simulink model "Model_TranslationEngine64"  (R2022b)
settings: Solver=FixedStepDiscrete  StartTime=0.0  StopTime=5  RelTol=1e-3  EnableMultiTasking=on
InitFcn:
  | % Initialize model
  | ModelSettings=BTConfig.GetModelSettings();
  | 
  | ModelSettings.Validate();
  | 
  | ModelInit;
  | 
  | 
  | % load library data
  | GainLibrary_data;
  | % Load saved values from partition process
  | CapturedConstMask.LoadMapFromFile(bdroot)
StartFcn:
  | % make sure all the simulated RTC requests are found
  | %RTC_SIM_OBJ.ValidateREQs();
undefined symbols (not defined in the file or in its folder): AA, BPLP, Column, NumHFRefBPF, NumHFRefLPF, NumMusicChannels, Row, VolumeMuteConfig
libraries: TuneVar x925, TOP x490, FeaturePath x111, CapturedConstLib x52
(part 14 of 34)

== system Model_TranslationEngine64/ModelPreAmp/DecRate/Medusa5H1/SleepingBeauty/SleepingBeauty/Enabled ==
  FadeControl : Subsystem  mask(Bose FadeControl){MaskIndexOffset=128, MaskBoostDisable=off, MaskSilentExtreme=on, BankNumber=0}
      mask prompts: MaskIndexOffset "Index Offset"; MaskBoostDisable "Disable Boost"; MaskSilentExtreme "Enable Silent Extreme"; BankNumber "Target Memory Bank Number"
      mask help: This component is to be used in conjunction with 1 or more instances of the FadeRamper block. It provides the control layer for Fade processing via an RTC and tune variables.
      mask init:
      | blkh = gcbh;
      | % Copy discrete mask parameters into a classdef object
      | InnerLinkConfig = FadeControlConfig;
      | InnerLinkConfig.DefaultIndexOffset = MaskIndexOffset;
      | InnerLinkConfig.DefaultBoostDisable = MaskBoostDisable;
      | InnerLinkConfig.DefaultSilentExtreme = MaskSilentExtreme;
      | InnerLinkConfig.BankNumber = BankNumber;
      mask Help: If this control block is being used in a "multi-instance" manner, i.e. it is contorlling two or more FadeRamper blocks, there is an additional step that must be done. The developer must add a function-triggered subsytem containing an AND logic gate, which will combine the notification completion signals of the multiple ramper instances. The output of this subsytem must then feed the NTF_done input of the FadeControl block.
  FadeRamperDR : Subsystem  mask(Bose FadeRamper){MaskFeatureName=FadeRamperDR, MaskChanRampMap=ones(1,30), MaskEnableGainPort=on}
      mask prompts: MaskFeatureName "Instance Name"; MaskChanRampMap "Channel to Ramper Map"; MaskEnableGainPort "Enable Output Gain Port"
      mask help:
      | This component is to be used in conjunction with the FadeControl block, which provides runtime control and tuning capabilities. Multiple instances of this block may be placed within an audio application, and a single FadeControl block has the ability to control all of these rampers simultaneously.
      |
      | For "Instance Name", please enter a name for the block. For example, if this is one of multiple instances of FadeRamper, then name each block accordingly so that the subsequent tune variables will route correctly.
      |
      | i.e. FadeRamper1, FadeRamper2, FadeRamperFullRate, etc.
      mask init:
      | blkh = gcbh;
      | % Copy discrete mask parameters into a classdef object
      | InnerLinkConfig = FadeRamperConfig;
      | InnerLinkConfig.DefaultChanRampMap = MaskChanRampMap;
      | 
      | % handle configurable output
      | EnableBlockPort(blkh,'fadeGains',MaskEnableGainPort,'2');
      mask TypeOptions MaskFeatureName: InnerLink/FeatureName
  FadeRamperFR : Subsystem  mask(Bose FadeRamper){MaskFeatureName=FadeRamperFR, MaskChanRampMap=ones(1,22), MaskEnableGainPort=on}
      mask prompts: MaskFeatureName "Instance Name"; MaskChanRampMap "Channel to Ramper Map"; MaskEnableGainPort "Enable Output Gain Port"
      mask help:
      | This component is to be used in conjunction with the FadeControl block, which provides runtime control and tuning capabilities. Multiple instances of this block may be placed within an audio application, and a single FadeControl block has the ability to control all of these rampers simultaneously.
      |
      | For "Instance Name", please enter a name for the block. For example, if this is one of multiple instances of FadeRamper, then name each block accordingly so that the subsequent tune variables will route correctly.
      |
      | i.e. FadeRamper1, FadeRamper2, FadeRamperFullRate, etc.
      mask init: same as Model_TranslationEngine64/ModelPreAmp/DecRate/Medusa5H1/SleepingBeauty/SleepingBeauty/Enabled/FadeRamperDR
      mask TypeOptions MaskFeatureName: InnerLink/FeatureName
  MuteControl : Subsystem  mask(Bose MuteControl){}
      mask help: This component is to be used in conjunction with 1 or more instances of the MuteRamper block. There is no mask for this component. It provides the control layer for Mute processing via an RTC and tune variable, muteControlRampTime.
      mask init:
      | InnerLinkConfig = MuteControlConfig;
      mask Help: If this control block is being used in a "multi-instance" manner, i.e. it is contorlling two or more MuteRamper blocks, there is an additional step that must be done. The developer must add a function-triggered subsytem containing an AND logic gate, which will combine the notification completion signals of the multiple ramper instances. The output of this subsytem must then feed the NTF_done input of the MuteControl block.
  SleepingBeautyDR : Subsystem  mask(Bose SleepingBeauty){MaskFeatureName=SleepingBeautyDR, MaskChanRampMap=ones(1,30), MaskOffset=128, MaskSilentExtremeMutesBass=off}
      mask prompts: MaskFeatureName "Instance Name"; MaskChanRampMap "Channel to Ramper Map"; MaskOffset "Control Index Offset"; MaskSilentExtremeMutesBass "Silent Extreme Mutes Bass"
      mask help:
      | This block is to be used in conjunction with the Balance block.
      |
      | For the Channel to Ramper Map, enter any of the following values:
      | 1 - left channel
      | 2 - right channel
      | 3 - center channel
      | 4 - mono channel
      | -1 - unused channel (will esentially be muted)
      | (For headrest speakers, choose a seat-centric ramper, i.e. Left Seat Left Ear and Left Seat Right Ear would both be considered "Left content", receiving a 1).
      |
      | Silent Extreme Mutes Bass: Check this box if the intention is for mono channels to be muted upon Silent Extreme
      |
      | If this block is being used in a multi-instance application, be sure to give independent names in each instance's mask.
      mask init:
      | blkh = gcbh;
      | % Copy discrete mask parameters into a classdef object
      | InnerLinkConfig = SleepingBeautyConfig;
      | InnerLinkConfig.ChanToRampMap = MaskChanRampMap;
      | InnerLinkConfig.DefaultOffset = MaskOffset;
      | InnerLinkConfig.DefaultSilentExtremeMutesBass = MaskSilentExtremeMutesBass;
      mask TypeOptions MaskFeatureName: InnerLink/FeatureName
  SleepingBeautyFR : Subsystem  mask(Bose SleepingBeauty){MaskFeatureName=SleepingBeautyFR, MaskChanRampMap=ones(1,22), MaskOffset=128, MaskSilentExtremeMutesBass=off}
      mask prompts: MaskFeatureName "Instance Name"; MaskChanRampMap "Channel to Ramper Map"; MaskOffset "Control Index Offset"; MaskSilentExtremeMutesBass "Silent Extreme Mutes Bass"
      mask help:
      | This block is to be used in conjunction with the Balance block.
      |
      | For the Channel to Ramper Map, enter any of the following values:
      | 1 - left channel
      | 2 - right channel
      | 3 - center channel
      | 4 - mono channel
      | -1 - unused channel (will esentially be muted)
      | (For headrest speakers, choose a seat-centric ramper, i.e. Left Seat Left Ear and Left Seat Right Ear would both be considered "Left content", receiving a 1).
      |
      | Silent Extreme Mutes Bass: Check this box if the intention is for mono channels to be muted upon Silent Extreme
      |
      | If this block is being used in a multi-instance application, be sure to give independent names in each instance's mask.
      mask init: same as Model_TranslationEngine64/ModelPreAmp/DecRate/Medusa5H1/SleepingBeauty/SleepingBeauty/Enabled/SleepingBeautyDR
      mask TypeOptions MaskFeatureName: InnerLink/FeatureName

== system Model_TranslationEngine64/ModelPreAmp/DecRate/Medusa5H1/VLS/Crosstalk Cancellation/Pooliir with Non-Trivial Translations ==
  InnerLink : Subsystem  mask(Bose Pool IIR Tunable){FeatureName=IIR, Config=InnerLinkConfig}
      mask prompts: FeatureName "Filter name/purpose"; Config "PoolIirTunableConfig"
      mask help:
      | Pool IIR Tunable is a configurable multi-channel IIR filter that supports one or more channels. This block offers flexibility of tuning the number of stages and coefficients. Different filter coefficients and number of stages (biquads) can be used for each channel filter. The Pool IIR Tunable block supports different implementations, which could be configured at build-time:
      |
      | (i)   Generic: IIR filter code not optimized for any processor
      | (ii)  SharcCore: IIR filters executing on core (uses pooliir.asm CRL)
      | (iii) SharcGulAccel: IIR filters executing on IIR hardware accelerator, offloading MIPS usage from core
      | (iv) SharcGxpAccel: IIR filters take advantage of additional accelerators available on GXP processor
      | (v)  Hexagon: TBD
      |
      | NOTE: When using Pool IIR for Sharc-plus based processors, the codeWorkMemory buffer and input buffer should always be mapped to L1 memory to optimize MIPS utilization and avoid audio artifacts.
      |
      | For more information, please see 'Help'.
      mask init:
      | blkh=gcbh;
      | Config=BTConfig.Assert(blkh,Config);
      | 
      | Config.Validate();
      | Config.DoMaskInit(blkh);
      mask Help:
      | <b>Input signals: </b>
      | AudioIn: input channels [frame size x number of channels]
      | 
      | <b>Output signals: </b>
      | AudioOut: output channels [frame size x number of channels]
      | 
      | <b>Mask parameters: </b>
      | PoolIirTunableConfig
      | Filter name/purpose
      mask TypeOptions FeatureName: PoolIirTunableWithReset/FeatureName
      mask Display: DrawPoolIirIcon;

== system Model_TranslationEngine64/ModelPreAmp/DecRate/Medusa5H1/VLS/Crosstalk Cancellation/TuneTOP ==
  TOP : TOP/TOP  TriggerInit=[440 20 585 80]  TopName=Delay  DataTypeOut=int32  BankNumber=BankNumber  PreOverlay=PreOverlay  PostOverlay=PostOverlay  Role=Automatic
      settings: SourceProductName=Bose Talaria
  TrivialTranslation : TuneVar/TrivialTranslation  TriggerInit=[300 28 350 72]
      settings: SourceProductName=Bose Talaria
  Tune Variable : TuneVar/TuneVar  TuneName=Delay  SpecifyMaxSize=off  VariableDim=1 (Row)  MaxSize=[1 1]  TunabilityNumber=1  MinValue=MinValue  MaxValue=MaxValue  TriggerInit=[20 25 190 75]  MaskValue=MaskValue
      settings: SourceProductName=Bose Talaria
  wires:
  Tune Variable/1 -> TrivialTranslation/1  "Delay"
  TrivialTranslation/1 -> TOP/1

== system Model_TranslationEngine64/ModelPreAmp/PreAmpPart1/NEARPreAmp/FixedAttenuator/Attenuation /Function-Call Subsystem ==
  In1 : Inport
  function : TriggerPort  TriggerType=function-call  VariantControl=Variant
  MATLAB Function : MATLAB Function  TreatAsAtomicUnit=on
  Out1 : Outport
  wires:
  MATLAB Function/1(lingain) -> Out1/1
  In1/1 -> MATLAB Function/1(dbgain)

== system Model_TranslationEngine64/ModelPreAmp/PreAmpPart1/NEARPreAmp/Monoizer/Monoizer/MonoizerStereo ==
  MonoizerCalc : Subsystem

== system Model_TranslationEngine64/ModelPreAmp/PreAmpPart1/NEARPreAmp/Monoizer/Monoizer/MonoizerSurround ==

== system Model_TranslationEngine64/NEAR/Near1p1/DrProc/FsEQDr/Pooliir/PoolIirTunableWithReset ==
  CapturedTuneConst : CapturedConstLib/CapturedConst  TriggerInit=[-600 302 -500 338]  Role=Automatic
      settings: SourceProductName=Bose Talaria
  FeaturePath : FeaturePath/FeaturePath  FeatureName=Pooliir  IsGroup=off  GroupNumber=-1  IsModule=off  TriggerInit=[-750 -81 -635 26]
      settings: SourceProductName=Bose Talaria
  TOP : TOP/TOP  TriggerInit=[-145 187 5 243]  TopName=PooliirNumStages  DataTypeOut=uint32  BankNumber=0  PreOverlay=false  PostOverlay=Config.VariantObj.PostOverlayRequired  Role=Automatic
      settings: SourceProductName=Bose Talaria
  TOP1 : TOP/TOP  TriggerInit=[-140 277 10 333]  TopName=pooliirCoeffs  DataTypeOut=single  BankNumber=0  PreOverlay=false  PostOverlay=Config.VariantObj.PostOverlayRequired  Role=Automatic
      settings: SourceProductName=Bose Talaria
  TranslateTrigger : TuneVar/TranslateTrigger  TriggerInit=[-339 35 -301 90]
      settings: SourceProductName=Bose Talaria
  Translation : MATLAB Function  TreatAsAtomicUnit=on  mask{MaxNumStages=Config.MaxNumStages, VariantUint8=Config.Variant.Uint8Str}
      mask prompts: VariantUint8 "Variant"
  Tune Variable1 : TuneVar/TuneVar  TuneName=numStages  SpecifyMaxSize=off  VariableDim=1 (Row)  MaxSize=[1 1]  TunabilityNumber=1  MinValue=[]  MaxValue=[]  TriggerInit=[-750 235 -580 285]  MaskValue=Config.TuneDefaults.NumStages
      settings: SourceProductName=Bose Talaria
  Tune Variable2 : TuneVar/TuneVar  TuneName=sosCoefficients  SpecifyMaxSize=on  VariableDim=1 (Row)  MaxSize=[Config.MaxNumStages 6]  TunabilityNumber=1  MinValue=[]  MaxValue=[]  TriggerInit=[-750 175 -580 225]  MaskValue=Config.TuneDefaults.SosCoefficients
      settings: SourceProductName=Bose Talaria
  wires:
  TranslateTrigger/1 -> Translation/Trigger
  Tune Variable2/1 -> Translation/1(RawSOS)  "sosCoefficients"
  Translation/2(PoolCoeffs) -> TOP1/1
  Translation/1(PoolNumStages) -> TOP/1
  Tune Variable1/1 -> Translation/2(NumStages)  "numStages"
  CapturedTuneConst/1 -> Translation/3(NumChannels)

== system Model_TranslationEngine64/NEAR/Near1p1/DrProc/FsEQDr/Subsystem1/Subsystem ==
  Tune Variable : TuneVar/TuneVar  TuneName=f1_del  SpecifyMaxSize=off  VariableDim=1 (Row)  MaxSize=[1 1]  TunabilityNumber=1  MinValue=[]  MaxValue=[]  TriggerInit=[20 20 190 70]  MaskValue=Config.f1_del
      settings: SourceProductName=Bose Talaria
  Tune Variable1 : TuneVar/TuneVar  TuneName=f2_del  SpecifyMaxSize=off  VariableDim=1 (Row)  MaxSize=[1 1]  TunabilityNumber=1  MinValue=[]  MaxValue=[]  TriggerInit=[20 155 190 205]  MaskValue=Config.f2_del
      settings: SourceProductName=Bose Talaria
  Tune Variable2 : TuneVar/TuneVar  TuneName=f3_del  SpecifyMaxSize=off  VariableDim=1 (Row)  MaxSize=[1 1]  TunabilityNumber=1  MinValue=[]  MaxValue=[]  TriggerInit=[20 290 190 340]  MaskValue=Config.f3_del
      settings: SourceProductName=Bose Talaria
  Tune Variable3 : TuneVar/TuneVar  TuneName=f4_del  SpecifyMaxSize=off  VariableDim=1 (Row)  MaxSize=[1 1]  TunabilityNumber=1  MinValue=[]  MaxValue=[]  TriggerInit=[20 425 190 475]  MaskValue=Config.f4_del
      settings: SourceProductName=Bose Talaria
  Tune Variable4 : TuneVar/TuneVar  TuneName=f5_del  SpecifyMaxSize=off  VariableDim=1 (Row)  MaxSize=[1 1]  TunabilityNumber=1  MinValue=[]  MaxValue=[]  TriggerInit=[20 560 190 610]  MaskValue=Config.f5_del
      settings: SourceProductName=Bose Talaria
  Tune Variable5 : TuneVar/TuneVar  TuneName=f6_del  SpecifyMaxSize=off  VariableDim=1 (Row)  MaxSize=[1 1]  TunabilityNumber=1  MinValue=[]  MaxValue=[]  TriggerInit=[20 695 190 745]  MaskValue=Config.f6_del
      settings: SourceProductName=Bose Talaria
  Tune Variable7 : TuneVar/TuneVar  TuneName=f7_del  SpecifyMaxSize=off  VariableDim=1 (Row)  MaxSize=[1 1]  TunabilityNumber=1  MinValue=[]  MaxValue=[]  TriggerInit=[20 825 190 875]  MaskValue=Config.f7_del
      settings: SourceProductName=Bose Talaria
  f1 : Outport
  f2 : Outport  Port=2
  f3 : Outport  Port=3
  f4 : Outport  Port=4
  f5 : Outport  Port=5
  f6 : Outport  Port=6
  f7 : Outport  Port=7
  wires:
  Tune Variable5/1 -> f6/1  "f6_del"
  Tune Variable2/1 -> f3/1  "f3_del"
  Tune Variable7/1 -> f7/1  "f7_del"
  Tune Variable/1 -> f1/1  "f1_del"
  Tune Variable1/1 -> f2/1  "f2_del"
  Tune Variable3/1 -> f4/1  "f4_del"
  Tune Variable4/1 -> f5/1  "f5_del"

== system Model_TranslationEngine64/NEAR/Near1p1/DrProc/HrEQDr/PoolIirTunable/PoolIirTunableWithReset ==
  CapturedTuneConst : CapturedConstLib/CapturedConst  TriggerInit=[-600 302 -500 338]  Role=Automatic
      settings: SourceProductName=Bose Talaria
  FeaturePath : FeaturePath/FeaturePath  FeatureName=PoolIirTunable  IsGroup=off  GroupNumber=-1  IsModule=off  TriggerInit=[-750 -81 -635 26]
      settings: SourceProductName=Bose Talaria
  TOP : TOP/TOP  TriggerInit=[-145 187 5 243]  TopName=PooliirNumStages  DataTypeOut=uint32  BankNumber=0  PreOverlay=false  PostOverlay=Config.VariantObj.PostOverlayRequired  Role=Automatic
      settings: SourceProductName=Bose Talaria
  TOP1 : TOP/TOP  TriggerInit=[-140 277 10 333]  TopName=pooliirCoeffs  DataTypeOut=single  BankNumber=0  PreOverlay=false  PostOverlay=Config.VariantObj.PostOverlayRequired  Role=Automatic
      settings: SourceProductName=Bose Talaria
  TranslateTrigger : TuneVar/TranslateTrigger  TriggerInit=[-339 35 -301 90]
      settings: SourceProductName=Bose Talaria
  Translation : MATLAB Function  TreatAsAtomicUnit=on  mask{MaxNumStages=Config.MaxNumStages, VariantUint8=Config.Variant.Uint8Str}
      mask prompts: VariantUint8 "Variant"
  Tune Variable1 : TuneVar/TuneVar  TuneName=numStages  SpecifyMaxSize=off  VariableDim=1 (Row)  MaxSize=[1 1]  TunabilityNumber=1  MinValue=[]  MaxValue=[]  TriggerInit=[-750 235 -580 285]  MaskValue=Config.TuneDefaults.NumStages
      settings: SourceProductName=Bose Talaria
  Tune Variable2 : TuneVar/TuneVar  TuneName=sosCoefficients  SpecifyMaxSize=on  VariableDim=1 (Row)  MaxSize=[Config.MaxNumStages 6]  TunabilityNumber=1  MinValue=[]  MaxValue=[]  TriggerInit=[-750 175 -580 225]  MaskValue=Config.TuneDefaults.SosCoefficients
      settings: SourceProductName=Bose Talaria
  wires:
  TranslateTrigger/1 -> Translation/Trigger
  Tune Variable2/1 -> Translation/1(RawSOS)  "sosCoefficients"
  Translation/2(PoolCoeffs) -> TOP1/1
  Translation/1(PoolNumStages) -> TOP/1
  Tune Variable1/1 -> Translation/2(NumStages)  "numStages"
  CapturedTuneConst/1 -> Translation/3(NumChannels)

== system Model_TranslationEngine64/NEAR/Near1p1/DrProc/HrEQDr/Subsystem2/Subsystem ==
  Tune Variable1 : TuneVar/TuneVar  TuneName=driver_src1  SpecifyMaxSize=off  VariableDim=1 (Row)  MaxSize=[1 1]  TunabilityNumber=1  MinValue=[]  MaxValue=[]  TriggerInit=[35 385 205 435]  MaskValue=Config.driver_src1
      settings: SourceProductName=Bose Talaria
  Tune Variable2 : TuneVar/TuneVar  TuneName=driver_src2  SpecifyMaxSize=off  VariableDim=1 (Row)  MaxSize=[1 1]  TunabilityNumber=1  MinValue=[]  MaxValue=[]  TriggerInit=[35 515 205 565]  MaskValue=Config.driver_src2
      settings: SourceProductName=Bose Talaria
  Tune Variable3 : TuneVar/TuneVar  TuneName=driver_src3  SpecifyMaxSize=off  VariableDim=1 (Row)  MaxSize=[1 1]  TunabilityNumber=1  MinValue=[]  MaxValue=[]  TriggerInit=[35 620 205 670]  MaskValue=Config.driver_src3
      settings: SourceProductName=Bose Talaria
  Tune Variable4 : TuneVar/TuneVar  TuneName=driver_src4  SpecifyMaxSize=off  VariableDim=1 (Row)  MaxSize=[1 1]  TunabilityNumber=1  MinValue=[]  MaxValue=[]  TriggerInit=[35 750 205 800]  MaskValue=Config.driver_src4
      settings: SourceProductName=Bose Talaria
  Tune Variable5 : TuneVar/TuneVar  TuneName=passenger_src1  SpecifyMaxSize=off  VariableDim=1 (Row)  MaxSize=[1 1]  TunabilityNumber=1  MinValue=[]  MaxValue=[]  TriggerInit=[35 880 205 930]  MaskValue=Config.passenger_src1
      settings: SourceProductName=Bose Talaria
  Tune Variable6 : TuneVar/TuneVar  TuneName=passenger_src3  SpecifyMaxSize=off  VariableDim=1 (Row)  MaxSize=[1 1]  TunabilityNumber=1  MinValue=[]  MaxValue=[]  TriggerInit=[35 1140 205 1190]  MaskValue=Config.passenger_src3
      settings: SourceProductName=Bose Talaria
  Tune Variable7 : TuneVar/TuneVar  TuneName=passenger_src2  SpecifyMaxSize=off  VariableDim=1 (Row)  MaxSize=[1 1]  TunabilityNumber=1  MinValue=[]  MaxValue=[]  TriggerInit=[35 1010 205 1060]  MaskValue=Config.passenger_src2
      settings: SourceProductName=Bose Talaria
  Tune Variable8 : TuneVar/TuneVar  TuneName=passenger_src4  SpecifyMaxSize=off  VariableDim=1 (Row)  MaxSize=[1 1]  TunabilityNumber=1  MinValue=[]  MaxValue=[]  TriggerInit=[30 1285 200 1335]  MaskValue=Config.passenger_src4
      settings: SourceProductName=Bose Talaria
  driver_src1 : Outport
  driver_src2 : Outport  Port=2
  driver_src3 : Outport  Port=3
  driver_src4 : Outport  Port=4
  passenger_src1 : Outport  Port=5
  passenger_src2 : Outport  Port=6
  passenger_src3 : Outport  Port=7
  passenger_src4 : Outport  Port=8
  wires:
  Tune Variable5/1 -> passenger_src1/1  "passenger_src1"
  Tune Variable7/1 -> passenger_src2/1  "passenger_src2"
  Tune Variable8/1 -> passenger_src4/1  "passenger_src4"
  Tune Variable6/1 -> passenger_src3/1  "passenger_src3"
  Tune Variable4/1 -> driver_src4/1  "driver_src4"
  Tune Variable3/1 -> driver_src3/1  "driver_src3"
  Tune Variable2/1 -> driver_src2/1  "driver_src2"
  Tune Variable1/1 -> driver_src1/1  "driver_src1"

== system Model_TranslationEngine64/NEAR/Near1p1/DrProc/Upmixer1p1Dr/Subsystem1/Subsystem ==
  Tune Variable : TuneVar/TuneVar  TuneName=f1_mix  SpecifyMaxSize=off  VariableDim=1 (Row)  MaxSize=[1 1]  TunabilityNumber=1  MinValue=[]  MaxValue=[]  TriggerInit=[20 20 190 70]  MaskValue=Config.TuneDefaults.f1_mix
      settings: SourceProductName=Bose Talaria
  Tune Variable1 : TuneVar/TuneVar  TuneName=f2_mix  SpecifyMaxSize=off  VariableDim=1 (Row)  MaxSize=[1 1]  TunabilityNumber=1  MinValue=[]  MaxValue=[]  TriggerInit=[20 155 190 205]  MaskValue=Config.TuneDefaults.f2_mix
      settings: SourceProductName=Bose Talaria
  Tune Variable2 : TuneVar/TuneVar  TuneName=f3_mix  SpecifyMaxSize=off  VariableDim=1 (Row)  MaxSize=[1 1]  TunabilityNumber=1  MinValue=[]  MaxValue=[]  TriggerInit=[20 290 190 340]  MaskValue=Config.TuneDefaults.f3_mix
      settings: SourceProductName=Bose Talaria
  Tune Variable3 : TuneVar/TuneVar  TuneName=f4_mix  SpecifyMaxSize=off  VariableDim=1 (Row)  MaxSize=[1 1]  TunabilityNumber=1  MinValue=[]  MaxValue=[]  TriggerInit=[20 425 190 475]  MaskValue=Config.TuneDefaults.f4_mix
      settings: SourceProductName=Bose Talaria
  Tune Variable4 : TuneVar/TuneVar  TuneName=f5_mix  SpecifyMaxSize=off  VariableDim=1 (Row)  MaxSize=[1 1]  TunabilityNumber=1  MinValue=[]  MaxValue=[]  TriggerInit=[20 560 190 610]  MaskValue=Config.TuneDefaults.f5_mix
      settings: SourceProductName=Bose Talaria
  Tune Variable5 : TuneVar/TuneVar  TuneName=f6_mix  SpecifyMaxSize=off  VariableDim=1 (Row)  MaxSize=[1 1]  TunabilityNumber=1  MinValue=[]  MaxValue=[]  TriggerInit=[20 695 190 745]  MaskValue=Config.TuneDefaults.f6_mix
      settings: SourceProductName=Bose Talaria
  Tune Variable7 : TuneVar/TuneVar  TuneName=f7_mix  SpecifyMaxSize=off  VariableDim=1 (Row)  MaxSize=[1 1]  TunabilityNumber=1  MinValue=[]  MaxValue=[]  TriggerInit=[20 825 190 875]  MaskValue=Config.TuneDefaults.f7_mix
      settings: SourceProductName=Bose Talaria
  f1 : Outport
  f2 : Outport  Port=2
  f3 : Outport  Port=3
  f4 : Outport  Port=4
  f5 : Outport  Port=5
  f6 : Outport  Port=6
  f7 : Outport  Port=7
  wires:
  Tune Variable5/1 -> f6/1  "f6_mix"
  Tune Variable2/1 -> f3/1  "f3_mix"
  Tune Variable7/1 -> f7/1  "f7_mix"
  Tune Variable/1 -> f1/1  "f1_mix"
  Tune Variable1/1 -> f2/1  "f2_mix"
  Tune Variable3/1 -> f4/1  "f4_mix"
  Tune Variable4/1 -> f5/1  "f5_mix"

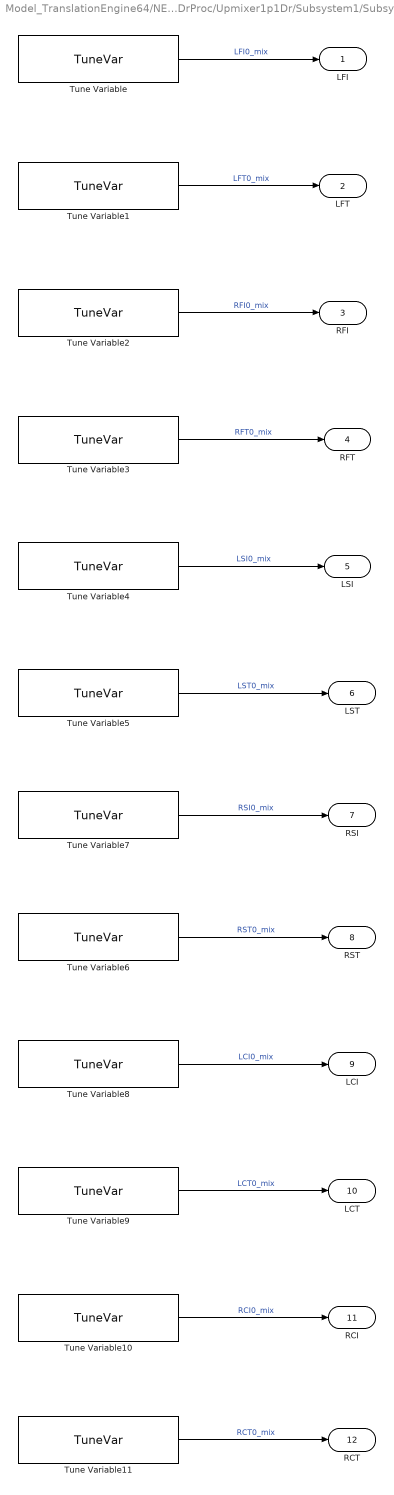
== system Model_TranslationEngine64/NEAR/Near1p1/DrProc/Upmixer1p1Dr/Subsystem1/Subsystem1 ==
  Tune Variable : TuneVar/TuneVar  TuneName=LFI0_mix  SpecifyMaxSize=off  VariableDim=1 (Row)  MaxSize=[1 1]  TunabilityNumber=1  MinValue=[]  MaxValue=[]  TriggerInit=[1315 -1070 1485 -1020]  MaskValue=Config.TuneDefaults.LFI0_mix
      settings: SourceProductName=Bose Talaria
  Tune Variable1 : TuneVar/TuneVar  TuneName=LFT0_mix  SpecifyMaxSize=off  VariableDim=1 (Row)  MaxSize=[1 1]  TunabilityNumber=1  MinValue=[]  MaxValue=[]  TriggerInit=[1315 -935 1485 -885]  MaskValue=Config.TuneDefaults.LFT0_mix
      settings: SourceProductName=Bose Talaria
  Tune Variable10 : TuneVar/TuneVar  TuneName=RCI0_mix  SpecifyMaxSize=off  VariableDim=1 (Row)  MaxSize=[1 1]  TunabilityNumber=1  MinValue=[]  MaxValue=[]  TriggerInit=[1315 270 1485 320]  MaskValue=Config.TuneDefaults.RCI0_mix
      settings: SourceProductName=Bose Talaria
  Tune Variable11 : TuneVar/TuneVar  TuneName=RCT0_mix  SpecifyMaxSize=off  VariableDim=1 (Row)  MaxSize=[1 1]  TunabilityNumber=1  MinValue=[]  MaxValue=[]  TriggerInit=[1315 400 1485 450]  MaskValue=Config.TuneDefaults.RCT0_mix
      settings: SourceProductName=Bose Talaria
  Tune Variable2 : TuneVar/TuneVar  TuneName=RFI0_mix  SpecifyMaxSize=off  VariableDim=1 (Row)  MaxSize=[1 1]  TunabilityNumber=1  MinValue=[]  MaxValue=[]  TriggerInit=[1315 -800 1485 -750]  MaskValue=Config.TuneDefaults.RFI0_mix
      settings: SourceProductName=Bose Talaria
  Tune Variable3 : TuneVar/TuneVar  TuneName=RFT0_mix  SpecifyMaxSize=off  VariableDim=1 (Row)  MaxSize=[1 1]  TunabilityNumber=1  MinValue=[]  MaxValue=[]  TriggerInit=[1315 -665 1485 -615]  MaskValue=Config.TuneDefaults.RFT0_mix
      settings: SourceProductName=Bose Talaria
  Tune Variable4 : TuneVar/TuneVar  TuneName=LSI0_mix  SpecifyMaxSize=off  VariableDim=1 (Row)  MaxSize=[1 1]  TunabilityNumber=1  MinValue=[]  MaxValue=[]  TriggerInit=[1315 -530 1485 -480]  MaskValue=Config.TuneDefaults.LSI0_mix
      settings: SourceProductName=Bose Talaria
  Tune Variable5 : TuneVar/TuneVar  TuneName=LST0_mix  SpecifyMaxSize=off  VariableDim=1 (Row)  MaxSize=[1 1]  TunabilityNumber=1  MinValue=[]  MaxValue=[]  TriggerInit=[1315 -395 1485 -345]  MaskValue=Config.TuneDefaults.LST0_mix
      settings: SourceProductName=Bose Talaria
  Tune Variable6 : TuneVar/TuneVar  TuneName=RST0_mix  SpecifyMaxSize=off  VariableDim=1 (Row)  MaxSize=[1 1]  TunabilityNumber=1  MinValue=[]  MaxValue=[]  TriggerInit=[1315 -135 1485 -85]  MaskValue=Config.TuneDefaults.RST0_mix
      settings: SourceProductName=Bose Talaria
  Tune Variable7 : TuneVar/TuneVar  TuneName=RSI0_mix  SpecifyMaxSize=off  VariableDim=1 (Row)  MaxSize=[1 1]  TunabilityNumber=1  MinValue=[]  MaxValue=[]  TriggerInit=[1315 -265 1485 -215]  MaskValue=Config.TuneDefaults.RSI0_mix
      settings: SourceProductName=Bose Talaria
  Tune Variable8 : TuneVar/TuneVar  TuneName=LCI0_mix  SpecifyMaxSize=off  VariableDim=1 (Row)  MaxSize=[1 1]  TunabilityNumber=1  MinValue=[]  MaxValue=[]  TriggerInit=[20 1090 190 1140]  MaskValue=Config.TuneDefaults.LCI0_mix
      settings: SourceProductName=Bose Talaria
  Tune Variable9 : TuneVar/TuneVar  TuneName=LCT0_mix  SpecifyMaxSize=off  VariableDim=1 (Row)  MaxSize=[1 1]  TunabilityNumber=1  MinValue=[]  MaxValue=[]  TriggerInit=[1315 135 1485 185]  MaskValue=Config.TuneDefaults.LCT0_mix
      settings: SourceProductName=Bose Talaria
  LFI : Outport
  LFT : Outport  Port=2
  RFI : Outport  Port=3
  RFT : Outport  Port=4
  LSI : Outport  Port=5
  LST : Outport  Port=6
  RSI : Outport  Port=7
  RST : Outport  Port=8
  LCI : Outport  Port=9
  LCT : Outport  Port=10
  RCI : Outport  Port=11
  RCT : Outport  Port=12
  wires:
  Tune Variable1/1 -> LFT/1  "LFT0_mix"
  Tune Variable11/1 -> RCT/1  "RCT0_mix"
  Tune Variable6/1 -> RST/1  "RST0_mix"
  Tune Variable3/1 -> RFT/1  "RFT0_mix"
  Tune Variable/1 -> LFI/1  "LFI0_mix"
  Tune Variable2/1 -> RFI/1  "RFI0_mix"
  Tune Variable7/1 -> RSI/1  "RSI0_mix"
  Tune Variable4/1 -> LSI/1  "LSI0_mix"
  Tune Variable8/1 -> LCI/1  "LCI0_mix"
  Tune Variable5/1 -> LST/1  "LST0_mix"
  Tune Variable9/1 -> LCT/1  "LCT0_mix"
  Tune Variable10/1 -> RCI/1  "RCI0_mix"

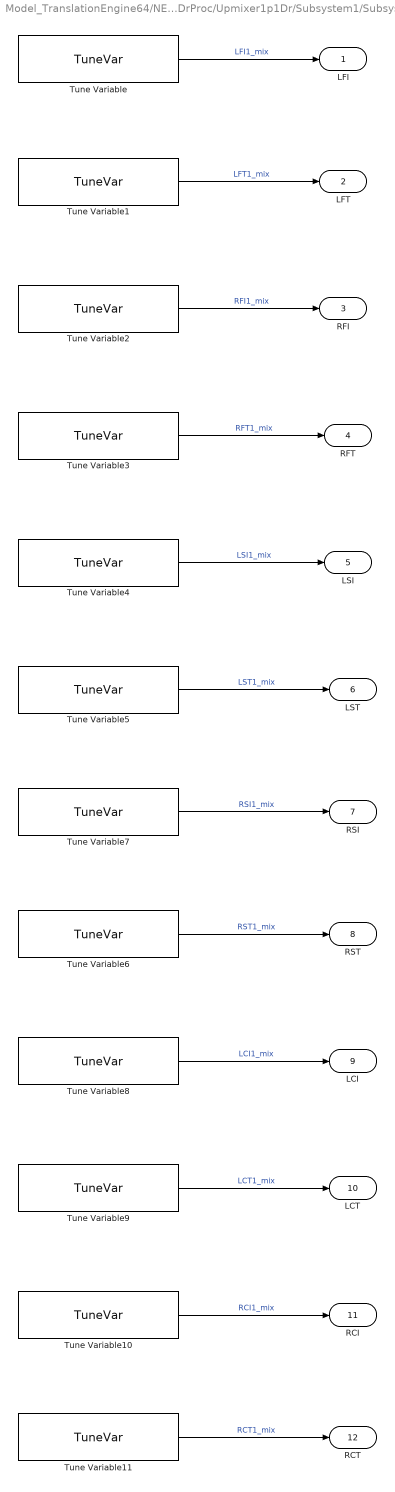
== system Model_TranslationEngine64/NEAR/Near1p1/DrProc/Upmixer1p1Dr/Subsystem1/Subsystem2 ==
  Tune Variable : TuneVar/TuneVar  TuneName=LFI1_mix  SpecifyMaxSize=off  VariableDim=1 (Row)  MaxSize=[1 1]  TunabilityNumber=1  MinValue=[]  MaxValue=[]  TriggerInit=[1315 910 1485 960]  MaskValue=Config.TuneDefaults.LFI1_mix
      settings: SourceProductName=Bose Talaria
  Tune Variable1 : TuneVar/TuneVar  TuneName=LFT1_mix  SpecifyMaxSize=off  VariableDim=1 (Row)  MaxSize=[1 1]  TunabilityNumber=1  MinValue=[]  MaxValue=[]  TriggerInit=[1315 1040 1485 1090]  MaskValue=Config.TuneDefaults.LFT1_mix
      settings: SourceProductName=Bose Talaria
  Tune Variable10 : TuneVar/TuneVar  TuneName=RCI1_mix  SpecifyMaxSize=off  VariableDim=1 (Row)  MaxSize=[1 1]  TunabilityNumber=1  MinValue=[]  MaxValue=[]  TriggerInit=[1315 2245 1485 2295]  MaskValue=Config.TuneDefaults.RCI1_mix
      settings: SourceProductName=Bose Talaria
  Tune Variable11 : TuneVar/TuneVar  TuneName=RCT1_mix  SpecifyMaxSize=off  VariableDim=1 (Row)  MaxSize=[1 1]  TunabilityNumber=1  MinValue=[]  MaxValue=[]  TriggerInit=[1315 2375 1485 2425]  MaskValue=Config.TuneDefaults.RCT1_mix
      settings: SourceProductName=Bose Talaria
  Tune Variable2 : TuneVar/TuneVar  TuneName=RFI1_mix  SpecifyMaxSize=off  VariableDim=1 (Row)  MaxSize=[1 1]  TunabilityNumber=1  MinValue=[]  MaxValue=[]  TriggerInit=[1315 1175 1485 1225]  MaskValue=Config.TuneDefaults.RFI1_mix
      settings: SourceProductName=Bose Talaria
  Tune Variable3 : TuneVar/TuneVar  TuneName=RFT1_mix  SpecifyMaxSize=off  VariableDim=1 (Row)  MaxSize=[1 1]  TunabilityNumber=1  MinValue=[]  MaxValue=[]  TriggerInit=[1315 1310 1485 1360]  MaskValue=Config.TuneDefaults.RFT1_mix
      settings: SourceProductName=Bose Talaria
  Tune Variable4 : TuneVar/TuneVar  TuneName=LSI1_mix  SpecifyMaxSize=off  VariableDim=1 (Row)  MaxSize=[1 1]  TunabilityNumber=1  MinValue=[]  MaxValue=[]  TriggerInit=[1315 1445 1485 1495]  MaskValue=Config.TuneDefaults.LSI1_mix
      settings: SourceProductName=Bose Talaria
  Tune Variable5 : TuneVar/TuneVar  TuneName=LST1_mix  SpecifyMaxSize=off  VariableDim=1 (Row)  MaxSize=[1 1]  TunabilityNumber=1  MinValue=[]  MaxValue=[]  TriggerInit=[1315 1580 1485 1630]  MaskValue=Config.TuneDefaults.LST1_mix
      settings: SourceProductName=Bose Talaria
  Tune Variable6 : TuneVar/TuneVar  TuneName=RST1_mix  SpecifyMaxSize=off  VariableDim=1 (Row)  MaxSize=[1 1]  TunabilityNumber=1  MinValue=[]  MaxValue=[]  TriggerInit=[1315 1840 1485 1890]  MaskValue=Config.TuneDefaults.RST1_mix
      settings: SourceProductName=Bose Talaria
  Tune Variable7 : TuneVar/TuneVar  TuneName=RSI1_mix  SpecifyMaxSize=off  VariableDim=1 (Row)  MaxSize=[1 1]  TunabilityNumber=1  MinValue=[]  MaxValue=[]  TriggerInit=[1315 1710 1485 1760]  MaskValue=Config.TuneDefaults.RSI1_mix
      settings: SourceProductName=Bose Talaria
  Tune Variable8 : TuneVar/TuneVar  TuneName=LCI1_mix  SpecifyMaxSize=off  VariableDim=1 (Row)  MaxSize=[1 1]  TunabilityNumber=1  MinValue=[]  MaxValue=[]  TriggerInit=[1315 1975 1485 2025]  MaskValue=Config.TuneDefaults.LCI1_mix
      settings: SourceProductName=Bose Talaria
  Tune Variable9 : TuneVar/TuneVar  TuneName=LCT1_mix  SpecifyMaxSize=off  VariableDim=1 (Row)  MaxSize=[1 1]  TunabilityNumber=1  MinValue=[]  MaxValue=[]  TriggerInit=[1315 2110 1485 2160]  MaskValue=Config.TuneDefaults.LCT1_mix
      settings: SourceProductName=Bose Talaria
  LFI : Outport
  LFT : Outport  Port=2
  RFI : Outport  Port=3
  RFT : Outport  Port=4
  LSI : Outport  Port=5
  LST : Outport  Port=6
  RSI : Outport  Port=7
  RST : Outport  Port=8
  LCI : Outport  Port=9
  LCT : Outport  Port=10
  RCI : Outport  Port=11
  RCT : Outport  Port=12
  wires:
  Tune Variable3/1 -> RFT/1  "RFT1_mix"
  Tune Variable/1 -> LFI/1  "LFI1_mix"
  Tune Variable7/1 -> RSI/1  "RSI1_mix"
  Tune Variable2/1 -> RFI/1  "RFI1_mix"
  Tune Variable4/1 -> LSI/1  "LSI1_mix"
  Tune Variable1/1 -> LFT/1  "LFT1_mix"
  Tune Variable11/1 -> RCT/1  "RCT1_mix"
  Tune Variable5/1 -> LST/1  "LST1_mix"
  Tune Variable6/1 -> RST/1  "RST1_mix"
  Tune Variable8/1 -> LCI/1  "LCI1_mix"
  Tune Variable9/1 -> LCT/1  "LCT1_mix"
  Tune Variable10/1 -> RCI/1  "RCI1_mix"

== system Model_TranslationEngine64/NEAR/Near1p1/DrProc/Upmixer1p1Dr/Subsystem1/Subsystem3 ==
  Tune Variable : TuneVar/TuneVar  TuneName=nv0l_mix  SpecifyMaxSize=off  VariableDim=1 (Row)  MaxSize=[1 1]  TunabilityNumber=1  MinValue=[]  MaxValue=[]  TriggerInit=[1345 730 1515 780]  MaskValue=Config.TuneDefaults.nv0l_mix
      settings: SourceProductName=Bose Talaria
  Tune Variable1 : TuneVar/TuneVar  TuneName=nv0r_mix  SpecifyMaxSize=off  VariableDim=1 (Row)  MaxSize=[1 1]  TunabilityNumber=1  MinValue=[]  MaxValue=[]  TriggerInit=[1345 865 1515 915]  MaskValue=Config.TuneDefaults.nv0r_mix
      settings: SourceProductName=Bose Talaria
  Tune Variable2 : TuneVar/TuneVar  TuneName=nv1l_mix  SpecifyMaxSize=off  VariableDim=1 (Row)  MaxSize=[1 1]  TunabilityNumber=1  MinValue=[]  MaxValue=[]  TriggerInit=[1345 1000 1515 1050]  MaskValue=Config.TuneDefaults.nv1l_mix
      settings: SourceProductName=Bose Talaria
  Tune Variable3 : TuneVar/TuneVar  TuneName=nv1r_mix  SpecifyMaxSize=off  VariableDim=1 (Row)  MaxSize=[1 1]  TunabilityNumber=1  MinValue=[]  MaxValue=[]  TriggerInit=[1345 1135 1515 1185]  MaskValue=Config.TuneDefaults.nv1r_mix
      settings: SourceProductName=Bose Talaria
  nv0l : Outport
  nv0r : Outport  Port=2
  nv1l : Outport  Port=3
  nv1r : Outport  Port=4
  wires:
  Tune Variable1/1 -> nv0r/1  "nv0r_mix"
  Tune Variable/1 -> nv0l/1  "nv0l_mix"
  Tune Variable3/1 -> nv1r/1  "nv1r_mix"
  Tune Variable2/1 -> nv1l/1  "nv1l_mix"

== system Model_TranslationEngine64/NEAR/Near1p1/FrProc/Subsystem/FsEQFr/Pooliir ==
  PoolIirTunableWithReset : Subsystem  mask(Bose Pool IIR Tunable){FeatureName=Pooliir, Config=Config}
      mask prompts: FeatureName "Filter name/purpose"; Config "PoolIirTunableWithResetConfig"
      mask help:
      | Pool IIR Tunable is a configurable multi-channel IIR filter that supports one or more channels. This block offers flexibility of tuning the number of stages and coefficients. Different filter coefficients and number of stages (biquads) can be used for each channel filter. The Pool IIR Tunable block supports different implementations, which could be configured at build-time:
      |
      | (i)   Generic: IIR filter code not optimized for any processor
      | (ii)  SharcCore: IIR filters executing on core (uses pooliir.asm CRL)
      | (iii) SharcGulAccel: IIR filters executing on IIR hardware accelerator, offloading MIPS usage from core
      | (iv) SharcGxpAccel: IIR filters take advantage of additional accelerators available on GXP processor
      | (v)  Hexagon: TBD
      |
      | NOTE: When using Pool IIR for Sharc-plus based processors, the codeWorkMemory buffer and input buffer should always be mapped to L1 memory to optimize MIPS utilization and avoid audio artifacts.
      |
      | For more information, please see 'Help'.
      mask init:
      | blkh=gcbh;
      | Config=BTConfig.Assert(blkh,Config);
      | 
      | BTConfig.InitSetFeatureIfPresent(blkh,'FeatureName');
      | Config.Validate();
      | Config.DoMaskInit(blkh);
      mask Help:
      | <b>Input signals: </b>
      | AudioIn: input channels [frame size x number of channels]
      | ResetTrigger: trigger to reset internal state buffer (usually preferred as a post RMDL step)
      | 
      | <b>Output signals: </b>
      | AudioOut: output channels [frame size x number of channels]
      | 
      | <b>Mask parameters: </b>
      | PoolIirTunableWithResetConfig
      | Filter name/purpose
      mask TypeOptions FeatureName: FeaturePath/FeatureName
      mask Callback Config: BTConfig.CallbackHideIfPresent(gcbh,{'FeatureName'});
      mask Display: DrawPoolIirIcon;

== system Model_TranslationEngine64/NEAR/Near1p1/FrProc/Subsystem/FsEQFr/Subsystem1 ==
  Subsystem : Subsystem
  TOP : TOP/TOP  TriggerInit=[275 30 420 90]  TopName=EqDelays  DataTypeOut=int32  BankNumber=0  PreOverlay=false  PostOverlay=false  Role=Automatic
      settings: SourceProductName=Bose Talaria
  TranslateTrigger : TuneVar/TranslateTrigger  TriggerInit=[-9 -280 29 -225]
      settings: SourceProductName=Bose Talaria
  Translation : MATLAB Function  TreatAsAtomicUnit=on
  wires:
  TranslateTrigger/1 -> Translation/Trigger
  Subsystem/7(f7) -> Translation/7(F7)
  Subsystem/3(f3) -> Translation/3(F3)
  Subsystem/1(f1) -> Translation/1(F1)
  Subsystem/2(f2) -> Translation/2(F2)
  Subsystem/4(f4) -> Translation/4(F4)
  Subsystem/5(f5) -> Translation/5(F5)
  Subsystem/6(f6) -> Translation/6(F6)
  Translation/1(eqdelays) -> TOP/1

== system Model_TranslationEngine64/NEAR/Near1p1/FrProc/Subsystem/HrEQFr/PoolIirTunable ==
  PoolIirTunableWithReset : Subsystem  mask(Bose Pool IIR Tunable){FeatureName=PoolIirTunable, Config=Config}
      mask prompts: FeatureName "Filter name/purpose"; Config "PoolIirTunableWithResetConfig"
      mask help:
      | Pool IIR Tunable is a configurable multi-channel IIR filter that supports one or more channels. This block offers flexibility of tuning the number of stages and coefficients. Different filter coefficients and number of stages (biquads) can be used for each channel filter. The Pool IIR Tunable block supports different implementations, which could be configured at build-time:
      |
      | (i)   Generic: IIR filter code not optimized for any processor
      | (ii)  SharcCore: IIR filters executing on core (uses pooliir.asm CRL)
      | (iii) SharcGulAccel: IIR filters executing on IIR hardware accelerator, offloading MIPS usage from core
      | (iv) SharcGxpAccel: IIR filters take advantage of additional accelerators available on GXP processor
      | (v)  Hexagon: TBD
      |
      | NOTE: When using Pool IIR for Sharc-plus based processors, the codeWorkMemory buffer and input buffer should always be mapped to L1 memory to optimize MIPS utilization and avoid audio artifacts.
      |
      | For more information, please see 'Help'.
      mask init:
      | blkh=gcbh;
      | Config=BTConfig.Assert(blkh,Config);
      | 
      | BTConfig.InitSetFeatureIfPresent(blkh,'FeatureName');
      | Config.Validate();
      | Config.DoMaskInit(blkh);
      mask Help:
      | <b>Input signals: </b>
      | AudioIn: input channels [frame size x number of channels]
      | ResetTrigger: trigger to reset internal state buffer (usually preferred as a post RMDL step)
      | 
      | <b>Output signals: </b>
      | AudioOut: output channels [frame size x number of channels]
      | 
      | <b>Mask parameters: </b>
      | PoolIirTunableWithResetConfig
      | Filter name/purpose
      mask TypeOptions FeatureName: FeaturePath/FeatureName
      mask Callback Config: BTConfig.CallbackHideIfPresent(gcbh,{'FeatureName'});
      mask Display: DrawPoolIirIcon;

== system Model_TranslationEngine64/NEAR/Near1p1/FrProc/Subsystem/HrEQFr/Subsystem2 ==
  Subsystem : Subsystem
  TOP : TOP/TOP  TriggerInit=[255 55 400 115]  TopName=eqdelays  DataTypeOut=single  BankNumber=0  PreOverlay=false  PostOverlay=false  Role=Automatic
      settings: SourceProductName=Bose Talaria
  TranslateTrigger : TuneVar/TranslateTrigger  TriggerInit=[-9 -280 29 -225]
      settings: SourceProductName=Bose Talaria
  Translation : MATLAB Function  TreatAsAtomicUnit=on  mask{NumHeadrestSpeakers=Config.NumHeadrestSpeakers, AnnChannelCount=Config.AnnChannelCount}
  wires:
  Subsystem/8(passenger_src4) -> Translation/8(passengersrc4)
  Subsystem/7(passenger_src3) -> Translation/7(passengersrc3)
  Subsystem/6(passenger_src2) -> Translation/6(passengersrc2)
  Subsystem/5(passenger_src1) -> Translation/5(passengersrc1)
  Subsystem/4(driver_src4) -> Translation/4(driversrc4)
  Subsystem/3(driver_src3) -> Translation/3(driversrc3)
  Subsystem/2(driver_src2) -> Translation/2(driversrc2)
  Subsystem/1(driver_src1) -> Translation/1(driversrc1)
  TranslateTrigger/1 -> Translation/Trigger
  Translation/1(eqdelays) -> TOP/1

== system Model_TranslationEngine64/NEAR/Near1p1/FrProc/Subsystem/RouterFr/InnerLink ==
  FeaturePath : FeaturePath/FeaturePath  FeatureName=Router  IsGroup=off  GroupNumber=-1  IsModule=off  TriggerInit=[615 164 730 271]
      settings: SourceProductName=Bose Talaria
  TOP : TOP/TOP  TriggerInit=[660 425 805 485]  TopName=OutMap  DataTypeOut=int32  BankNumber=0  PreOverlay=false  PostOverlay=false  Role=Automatic
      settings: SourceProductName=Bose Talaria
  TranslateTrigger : TuneVar/TranslateTrigger  TriggerInit=[526 305 564 360]
      settings: SourceProductName=Bose Talaria
  Trivial Translation : MATLAB Function  TreatAsAtomicUnit=on  mask{nInRouterMask=Config.NumIn}
      mask prompts: nInRouterMask "Num Input"
  TuneVarRouterMap : TuneVar/TuneVar  TuneName=Map  SpecifyMaxSize=on  VariableDim=2 (Column)  MaxSize=[1 Config.NumOut]  TunabilityNumber=1  MinValue=[]  MaxValue=[]  TriggerInit=[250 430 420 480]  MaskValue=Config.DefaultOutputMap
      settings: SourceProductName=Bose Talaria
  wires:
  TranslateTrigger/1 -> Trivial Translation/Trigger
  Trivial Translation/1(OutMap) -> TOP/1
  TuneVarRouterMap/1 -> Trivial Translation/1(Map)  "Map"

== system Model_TranslationEngine64/NEAR/Near1p1/FrProc/Subsystem/Upmixer1p1Fr/Subsystem1 ==
  Subsystem : Subsystem
  Subsystem1 : Subsystem
  Subsystem2 : Subsystem
  Subsystem3 : Subsystem
  TOP : TOP/TOP  TriggerInit=[2060 145 2205 205]  TopName=mix  DataTypeOut=single  BankNumber=0  PreOverlay=false  PostOverlay=false  Role=Automatic
      settings: SourceProductName=Bose Talaria
  TranslateTrigger : TuneVar/TranslateTrigger  TriggerInit=[1811 -585 1849 -530]
      settings: SourceProductName=Bose Talaria
  Translation : MATLAB Function  TreatAsAtomicUnit=on  mask{FrontPeripheralChannelCount=Config.FrontPeripheralChannelCount, HeadrestCount=Config.HeadrestCount, ChannelsPerHeadrest=Config.ChannelsPerHeadrest}
  wires:
  Subsystem3/4(nv1r) -> Translation/35(nv1r)
  Subsystem3/3(nv1l) -> Translation/34(nv1l)
  Subsystem3/2(nv0r) -> Translation/33(nv0r)
  Subsystem3/1(nv0l) -> Translation/32(nv0l)
  Translation/1(mix) -> TOP/1
  Subsystem2/1(LFI) -> Translation/20(LFI1)
  Subsystem2/2(LFT) -> Translation/21(LFT1)
  Subsystem2/3(RFI) -> Translation/22(RFI1)
  Subsystem2/4(RFT) -> Translation/23(RFT1)
  Subsystem2/5(LSI) -> Translation/24(LSI1)
  Subsystem2/6(LST) -> Translation/25(LST1)
  Subsystem2/7(RSI) -> Translation/26(RSI1)
  Subsystem2/8(RST) -> Translation/27(RST1)
  Subsystem2/9(LCI) -> Translation/28(LCI1)
  Subsystem2/10(LCT) -> Translation/29(LCT1)
  Subsystem2/11(RCI) -> Translation/30(RCI1)
  Subsystem2/12(RCT) -> Translation/31(RCT1)
  Subsystem/7(f7) -> Translation/7(F7)
  Subsystem/6(f6) -> Translation/6(F6)
  Subsystem/5(f5) -> Translation/5(F5)
  Subsystem/4(f4) -> Translation/4(F4)
  Subsystem/3(f3) -> Translation/3(F3)
  Subsystem/2(f2) -> Translation/2(F2)
  Subsystem/1(f1) -> Translation/1(F1)
  Subsystem1/12(RCT) -> Translation/19(RCT0)
  Subsystem1/11(RCI) -> Translation/18(RCI0)
  Subsystem1/10(LCT) -> Translation/17(LCT0)
  Subsystem1/9(LCI) -> Translation/16(LCI0)
  Subsystem1/8(RST) -> Translation/15(RST0)
  Subsystem1/7(RSI) -> Translation/14(RSI0)
  Subsystem1/6(LST) -> Translation/13(LST0)
  Subsystem1/5(LSI) -> Translation/12(LSI0)
  Subsystem1/4(RFT) -> Translation/11(RFT0)
  Subsystem1/3(RFI) -> Translation/10(RFI0)
  Subsystem1/2(LFT) -> Translation/9(LFT0)
  Subsystem1/1(LFI) -> Translation/8(LFI0)
  TranslateTrigger/1 -> Translation/Trigger

== system Model_TranslationEngine64/NEAR/Near1p1/VolumeMute/AnnouncementLevelDetector/PreProcessing/PreEmphasisShelfFilter ==
  PoolIirTunableWithReset : Subsystem  mask(Bose Pool IIR Tunable){FeatureName=PreEmphasisShelfFilter, Config=Config}
      mask prompts: FeatureName "Filter name/purpose"; Config "PoolIirTunableWithResetConfig"
      mask help:
      | Pool IIR Tunable is a configurable multi-channel IIR filter that supports one or more channels. This block offers flexibility of tuning the number of stages and coefficients. Different filter coefficients and number of stages (biquads) can be used for each channel filter. The Pool IIR Tunable block supports different implementations, which could be configured at build-time:
      |
      | (i)   Generic: IIR filter code not optimized for any processor
      | (ii)  SharcCore: IIR filters executing on core (uses pooliir.asm CRL)
      | (iii) SharcGulAccel: IIR filters executing on IIR hardware accelerator, offloading MIPS usage from core
      | (iv) SharcGxpAccel: IIR filters take advantage of additional accelerators available on GXP processor
      | (v)  Hexagon: TBD
      |
      | NOTE: When using Pool IIR for Sharc-plus based processors, the codeWorkMemory buffer and input buffer should always be mapped to L1 memory to optimize MIPS utilization and avoid audio artifacts.
      |
      | For more information, please see 'Help'.
      mask init:
      | blkh=gcbh;
      | Config=BTConfig.Assert(blkh,Config);
      | 
      | BTConfig.InitSetFeatureIfPresent(blkh,'FeatureName');
      | Config.Validate();
      | Config.DoMaskInit(blkh);
      mask Help:
      | <b>Input signals: </b>
      | AudioIn: input channels [frame size x number of channels]
      | ResetTrigger: trigger to reset internal state buffer (usually preferred as a post RMDL step)
      | 
      | <b>Output signals: </b>
      | AudioOut: output channels [frame size x number of channels]
      | 
      | <b>Mask parameters: </b>
      | PoolIirTunableWithResetConfig
      | Filter name/purpose
      mask TypeOptions FeatureName: FeaturePath/FeatureName
      mask Callback Config: BTConfig.CallbackHideIfPresent(gcbh,{'FeatureName'});
      mask Display: DrawPoolIirIcon;

== system Model_TranslationEngine64/NEAR/Near1p1/VolumeMute/AnnouncementLevelDetector/PreProcessing/sys_max_dbspl ==
  TOP : TOP/TOP  TriggerInit=[440 20 585 80]  TopName=SysMaxDbspl  DataTypeOut=single  BankNumber=BankNumber  PreOverlay=PreOverlay  PostOverlay=PostOverlay  Role=Automatic
      settings: SourceProductName=Bose Talaria
  TrivialTranslation : TuneVar/TrivialTranslation  TriggerInit=[300 28 350 72]
      settings: SourceProductName=Bose Talaria
  Tune Variable : TuneVar/TuneVar  TuneName=SysMaxDbspl  SpecifyMaxSize=off  VariableDim=1 (Row)  MaxSize=[1 1]  TunabilityNumber=1  MinValue=MinValue  MaxValue=MaxValue  TriggerInit=[20 25 190 75]  MaskValue=MaskValue
      settings: SourceProductName=Bose Talaria
  wires:
  Tune Variable/1 -> TrivialTranslation/1  "SysMaxDbspl"
  TrivialTranslation/1 -> TOP/1

== system Model_TranslationEngine64/NEAR/Near1p1/VolumeMute/AnnouncementLevelDetector/ch1_level/fast_decay ==
  TOP : TOP/TOP  TriggerInit=[415 20 675 80]  TopName=FastDecayDbPerSample  DataTypeOut=Inherit: Same as input  BankNumber=0  PreOverlay=false  PostOverlay=false  Role=Automatic
      settings: SourceProductName=Bose Talaria
  TranslateTrigger : TuneVar/TranslateTrigger  TriggerInit=[291 -100 329 -45]
      settings: SourceProductName=Bose Talaria
  Tune Variable : TuneVar/TuneVar  TuneName=FastDecayDbPers  SpecifyMaxSize=off  VariableDim=1 (Row)  MaxSize=[1 1]  TunabilityNumber=1  MinValue=[]  MaxValue=[]  TriggerInit=[-135 20 125 80]  MaskValue=Config.DefaultAnn1LevelDetectFastDecayDbPers
      settings: SourceProductName=Bose Talaria
  sec2samples : MATLAB Function  TreatAsAtomicUnit=on  mask{FrameRate=Config.FrameRate}
  wires:
  TranslateTrigger/1 -> sec2samples/Trigger
  sec2samples/1(y) -> TOP/1
  Tune Variable/1 -> sec2samples/1(u)  "FastDecayDbPers"

== system Model_TranslationEngine64/NEAR/Near1p1/VolumeMute/AnnouncementLevelDetector/ch1_level/hold_margin ==
  SetPositive : MATLAB Function  TreatAsAtomicUnit=on
  TOP : TOP/TOP  TriggerInit=[440 20 640 80]  TopName=hold_margin_db  DataTypeOut=single  BankNumber=0  PreOverlay=false  PostOverlay=false  Role=Automatic
      settings: SourceProductName=Bose Talaria
  TranslateTrigger : TuneVar/TranslateTrigger  TriggerInit=[306 -100 344 -45]
      settings: SourceProductName=Bose Talaria
  Tune Variable : TuneVar/TuneVar  TuneName=HoldMarginDb  SpecifyMaxSize=off  VariableDim=1 (Row)  MaxSize=[1 1]  TunabilityNumber=1  MinValue=[]  MaxValue=[]  TriggerInit=[-120 22 90 78]  MaskValue=Config.DefaultAnn1LevelDetectHoldMarginDb
      settings: SourceProductName=Bose Talaria
  wires:
  TranslateTrigger/1 -> SetPositive/Trigger
  SetPositive/1(TOP) -> TOP/1
  Tune Variable/1 -> SetPositive/1(Tune)  "HoldMarginDb"

== system Model_TranslationEngine64/NEAR/Near1p1/VolumeMute/AnnouncementLevelDetector/ch1_level/hold_time ==
  TOP : TOP/TOP  TriggerInit=[495 17 755 83]  TopName=HoldTimeSamples  DataTypeOut=Inherit: Same as input  BankNumber=0  PreOverlay=false  PostOverlay=false  Role=Automatic
      settings: SourceProductName=Bose Talaria
  TranslateTrigger : TuneVar/TranslateTrigger  TriggerInit=[306 -100 344 -45]
      settings: SourceProductName=Bose Talaria
  Tune Variable : TuneVar/TuneVar  TuneName=HoldTimes  SpecifyMaxSize=off  VariableDim=1 (Row)  MaxSize=[1 1]  TunabilityNumber=1  MinValue=[]  MaxValue=[]  TriggerInit=[-95 17 165 83]  MaskValue=Config.DefaultAnn1LevelDetectHoldTimes
      settings: SourceProductName=Bose Talaria
  sec2samples : MATLAB Function  TreatAsAtomicUnit=on  mask{FrameRate=Config.FrameRate}
  wires:
  TranslateTrigger/1 -> sec2samples/Trigger
  sec2samples/1(y) -> TOP/1
  Tune Variable/1 -> sec2samples/1(u)  "HoldTimes"

== system Model_TranslationEngine64/NEAR/Near1p1/VolumeMute/AnnouncementLevelDetector/ch1_level/max_volume ==
  TOP : TOP/TOP  TriggerInit=[440 20 585 80]  TopName=MaxVolumeDb  DataTypeOut=single  BankNumber=BankNumber  PreOverlay=PreOverlay  PostOverlay=PostOverlay  Role=Automatic
      settings: SourceProductName=Bose Talaria
  TrivialTranslation : TuneVar/TrivialTranslation  TriggerInit=[300 28 350 72]
      settings: SourceProductName=Bose Talaria
  Tune Variable : TuneVar/TuneVar  TuneName=MaxVolumeDb  SpecifyMaxSize=off  VariableDim=1 (Row)  MaxSize=[1 1]  TunabilityNumber=1  MinValue=MinValue  MaxValue=MaxValue  TriggerInit=[20 25 190 75]  MaskValue=MaskValue
      settings: SourceProductName=Bose Talaria
  wires:
  Tune Variable/1 -> TrivialTranslation/1  "MaxVolumeDb"
  TrivialTranslation/1 -> TOP/1

== system Model_TranslationEngine64/NEAR/Near1p1/VolumeMute/AnnouncementLevelDetector/ch1_level/min_volume ==
  TOP : TOP/TOP  TriggerInit=[440 20 585 80]  TopName=MinVolumeDb  DataTypeOut=single  BankNumber=BankNumber  PreOverlay=PreOverlay  PostOverlay=PostOverlay  Role=Automatic
      settings: SourceProductName=Bose Talaria
  TrivialTranslation : TuneVar/TrivialTranslation  TriggerInit=[300 28 350 72]
      settings: SourceProductName=Bose Talaria
  Tune Variable : TuneVar/TuneVar  TuneName=MinVolumeDb  SpecifyMaxSize=off  VariableDim=1 (Row)  MaxSize=[1 1]  TunabilityNumber=1  MinValue=MinValue  MaxValue=MaxValue  TriggerInit=[20 25 190 75]  MaskValue=MaskValue
      settings: SourceProductName=Bose Talaria
  wires:
  Tune Variable/1 -> TrivialTranslation/1  "MinVolumeDb"
  TrivialTranslation/1 -> TOP/1

== system Model_TranslationEngine64/NEAR/Near1p1/VolumeMute/AnnouncementLevelDetector/ch1_level/slow_decay ==
  TOP : TOP/TOP  TriggerInit=[445 15 710 85]  TopName=SlowDecayDbPerSample  DataTypeOut=Inherit: Same as input  BankNumber=0  PreOverlay=false  PostOverlay=false  Role=Automatic
      settings: SourceProductName=Bose Talaria
  TranslateTrigger : TuneVar/TranslateTrigger  TriggerInit=[306 -100 344 -45]
      settings: SourceProductName=Bose Talaria
  Tune Variable : TuneVar/TuneVar  TuneName=SlowDecayDbPers  SpecifyMaxSize=off  VariableDim=1 (Row)  MaxSize=[1 1]  TunabilityNumber=1  MinValue=[]  MaxValue=[]  TriggerInit=[-115 15 150 85]  MaskValue=Config.DefaultAnn1LevelDetectSlowDecayDbPers
      settings: SourceProductName=Bose Talaria
  sec2samples : MATLAB Function  TreatAsAtomicUnit=on  mask{FrameRate=Config.FrameRate}
  wires:
  TranslateTrigger/1 -> sec2samples/Trigger
  sec2samples/1(y) -> TOP/1
  Tune Variable/1 -> sec2samples/1(u)  "SlowDecayDbPers"

== system Model_TranslationEngine64/NEAR/Near1p1/VolumeMute/AnnouncementLevelDetector/ch2_level/fast_decay ==
  TOP : TOP/TOP  TriggerInit=[495 17 745 83]  TopName=FastDecayDbPerSample  DataTypeOut=Inherit: Same as input  BankNumber=0  PreOverlay=false  PostOverlay=false  Role=Automatic
      settings: SourceProductName=Bose Talaria
  TranslateTrigger : TuneVar/TranslateTrigger  TriggerInit=[306 -100 344 -45]
      settings: SourceProductName=Bose Talaria
  Tune Variable : TuneVar/TuneVar  TuneName=FastDecayDbPers  SpecifyMaxSize=off  VariableDim=1 (Row)  MaxSize=[1 1]  TunabilityNumber=1  MinValue=[]  MaxValue=[]  TriggerInit=[-140 17 110 83]  MaskValue=Config.DefaultAnn2LevelDetectFastDecayDbPers
      settings: SourceProductName=Bose Talaria
  sec2samples : MATLAB Function  TreatAsAtomicUnit=on  mask{FrameRate=Config.FrameRate}
  wires:
  TranslateTrigger/1 -> sec2samples/Trigger
  sec2samples/1(y) -> TOP/1  "sec2samples"
  Tune Variable/1 -> sec2samples/1(u)  "FastDecayDbPers"
